simulink model "Sim_Multi"  (R2023a)
settings: Solver=FixedStepAuto  StartTime=0.0  StopTime=20  FixedStep=t_sim  MaxStep=t_control  RelTol=1e-5  EnableMultiTasking=on
InitFcn:
  | %--------------------------------------------------------------------------
  | %% Multirotor Dynamic Simulation Environment for the Testing of GNC Algorithms
  | % This simulation is part of the Master's thesis titled
  | % "A Modular Simulation Environment for the Improved Dynamic Simulation of
  | % Multirotor Unmanned Aerial Vehicles",
  | % submitted to the University of Illinois at Urbana-Champaign in May 2016.
  | % The thesis itself can be found here: http://hdl.handle.net/2142/90660
  | % Jan Vervoorst, vervoors@illinois.edu
  | % University of Illinois 2015/16
  | %--------------------------------------------------------------------------
  | %% Initialization routine for the Simulink simulation file Sim_Multi.slx
  | %--------------------------------------------------------------------------
  | clear all;close all;clc
  | %--------------------------------------------------------------------------
  | t_control = 1/500;          % Controller/state estimation frequency 500Hz [s]
  | t_sim = t_control/2;        % Simulation frequency 1000Hz [s]
  | sim_time = 10.0;            % Duration of simulation [sec]
  | r2d = 180/pi;               % Conversion factor radians to degrees [deg/rad]
  | d2r = pi/180;               % Conversion factor degrees to radians [rad/deg]
  | g = 9.80665;                % Acceleration of gravity [m/s^2]
  | rpm2radpersec = 2*pi/60;    % Conversion factor RPM to rad/sec [rad/(s*rpm)]
  | rho = 1.225;                % Density of air [kg/m^3]
  | %--------------------------------------------------------------------------
  | %%%%%%%%%%%%%%%%%%%%%%%%%%%%%%%%%%%%%%%%%%%%%%%%%%%%%%%%%%%%%%%%%%%%%%%%%%%
  | %               Quad specific configuration parameters                    %
  | %%%%%%%%%%%%%%%%%%%%%%%%%%%%%%%%%%%%%%%%%%%%%%%%%%%%%%%%%%%%%%%%%%%%%%%%%%%
  | % The coordinate system used in this model is defined as follows:
  | % X: pointing forward, Roll axis
  | % Y: pointing to the right, Pitch axis
  | % Z: pointing down, Yaw axis
  | % To define the geometry of the airframe, the following convention is used:
  | % - the base airframe is assumed to be somewhat symmetric
  | % - the CoG for the base airframe coincides with the geometric center in X/Y plane (but is shifted along Z axis)
  | % - the motor arm length in X/Y plane is defined as the distance to the geometric center of the base airframe
  | % - motor thrust is generated at the prop, which is offset a distance (along Z) from the geometric center
  | % - motor thrust vector may be misaligned from purely Z direction, so a set of rotation angles is given for each motor
  | % - real position of CoG is given as a position vector from geometric center
  | % - everything is expressed in body coordinate system described above
  | %%%%%%%%%%%%%%%%%%%%%%%%%%%%%%%%%%%%%%%%%%%%%%%%%%%%%%%%%%%%%%%%%%%%%%%%%%%
  | Noise_flag = 0;                 % Set to 1 for sensor/estimation noise, to 0 for no noise
  | Coriolis_correction = 1;        % Set to 1 to cancel omega x (J*omega) term in control law, 0 if not
  | Dyn_thrust = 1;                 % Set to 1 to engage dynamic thrust effects, to 0 to disengage
  | Blade_flapping = 1;             % Set to 1 to engage blade flapping effects, to 0 to disengage
  | %%%%%%%%%%%%%%%%%%%%%%%%%%%%%%%%
  | % Initial conditions
  | Att_init = [0;0;0] * d2r;       % Initial airframe attitude in Euler angles Roll/Pitch/Yaw for 6DOF block [deg]
  | omega_init = [0;0;0];           % Initial angular rates in Body frame for 6DOF block [rad/s]
  | Vb_init = [0;0;0];              % Initial velocity in Body frame for 6DOF block [m/s]
  | Xi_init = [0;0;0];              % Initial position in Inertial frame for 6DOF block [m]
  | rpm_init = 3104.5025852;        % Initial motor speed [rpm]
  | q_init = rpy2quat(Att_init);    % Compute the initial attitude quaternion
  | R_IB_init = rpy2rot(Att_init);  % Compute the initial rotation matrix R_IB
  | Vi_init = R_IB_init' * Vb_init; % Compute the initial velocity in Inertial axes
  | %%%%%%%%%%%%%%%%%%%%%%%%%%%%%%%%
  | % Parameters for aerodynamic drag computation
  | a = 0.060;                      % Surface area of airframe visible along the Body x axis [m^2]
  | b = 0.060;                      % Surface area of airframe visible along the Body y axis [m^2]
  | c = 0.060;                      % Surface area of airframe visible along the Body z axis [m^2]
  | C_D = 0.40;                     % Drag coefficient [dimensionless]
  | Surface_params = [a;b;c];       % Combine the surface area parameters
  | ... (+145 lines)
undefined symbols (not defined in the file or in its folder): DiscIntNeverNeededParam, rpy2quat, thrust2rpm
libraries: simulink x20
(part 4 of 4)

== system Sim_Multi/multirotor/Force//Moment computation/Forces and moments generated by spinning propellers/For Each Subsystem/Thrust//moment vector for each propeller (Body axes)/Compute dynamic motor thrust and moments/Dynamic thrust ratio/Flight modes of the propeller ==
  v_h : Inport
  v_c : Inport  Port=2
  Divide : Product  Inputs=*/  SampleTime=t_sim
  If : If  IfExpression=u1 >= 0  ElseIfExpressions=u1 >= -2  SampleTime=t_sim
  Merge : Merge  Inputs=3
  Normal working state vc/vh >= 0 : Subsystem  TreatAsAtomicUnit=on
  "Vortex ring state -2 <= vc/vh < 0 " : Subsystem  TreatAsAtomicUnit=on
  Windmill braking state vc/vh < -2 : Subsystem  TreatAsAtomicUnit=on
  v_i : Outport
  wires:
  Merge/1 -> v_i/1
  v_c/1 -> Windmill braking state vc/vh < -2/1(v_c), "Vortex ring state -2 <= vc/vh < 0 "/1(v_c), Normal working state vc/vh >= 0/1(v_c), Divide/1
  v_h/1 -> Divide/2
  Divide/1 -> If/1  "v_c/v_h"
  If/1 -> Normal working state vc/vh >= 0/Action
  Normal working state vc/vh >= 0/1(v_i) -> Merge/1
  "Vortex ring state -2 <= vc/vh < 0 "/1(v_i) -> Merge/2
  Windmill braking state vc/vh < -2/1(v_i) -> Merge/3
  If/2 -> "Vortex ring state -2 <= vc/vh < 0 "/Action
  If/3 -> Windmill braking state vc/vh < -2/Action

== system Sim_Multi/multirotor/Force//Moment computation/Forces and moments generated by spinning propellers/For Each Subsystem/Thrust//moment vector for each propeller (Body axes)/Compute dynamic motor thrust and moments/Gyroscopic torque/Cross Product ==
  u : Inport
  v : Inport  Port=2
  Subsystem : Subsystem
  Subsystem1 : Subsystem
  Sum : Sum  Inputs=+|-
  u x v : Outport
  wires:
  Sum/1 -> u x v/1
  u/1 -> Subsystem1/1(u), Subsystem/1(u)
  v/1 -> Subsystem1/2(v), Subsystem/2(v)
  Subsystem/1(Positive elements) -> Sum/1
  Subsystem1/1(Negative elements) -> Sum/2

== system Sim_Multi/multirotor/Force//Moment computation/Forces and moments generated by spinning propellers/For Each Subsystem/Thrust//moment vector for each propeller (Body axes)/Compute dynamic motor thrust and moments/Gyroscopic torque/Propeller moment of inertia ==
  note: This computes the approximate moment of inertia of a propeller given its mass and diameter.
      | It is the mean value of the disk approximation and the rod approximation for a spinning propeller.
  In1 : Inport
  Gain : Gain  Gain=0.5
  Gain1 : Gain  Gain=7/12
  Product7 : Product  Inputs=3
  Selector4 : Selector  InputPortWidth=17  IndexOptions=Index vector (dialog)  Indices=[16]  OutputSizes=1
  Selector5 : Selector  InputPortWidth=17  IndexOptions=Index vector (dialog)  Indices=[17]  OutputSizes=1
  Out1 : Outport
  wires:
  Selector5/1 -> Product7/3  "Propeller mass"
  Gain/1 -> Product7/2, Product7/1
  In1/1 -> Selector5/1, Selector4/1
  Selector4/1 -> Gain/1  "Propeller diameter"
  Gain1/1 -> Out1/1
  Product7/1 -> Gain1/1

== system Sim_Multi/multirotor/Force//Moment computation/Forces and moments generated by spinning propellers/For Each Subsystem/Thrust//moment vector for each propeller (Body axes)/Coordinate transformation Body to Motor axes/Rotation Matrix Body to Motor/Subsystem ==
  Euler : Inport
  Demux : Demux  Outputs=3
  Product : Product
  Terminator : Terminator
  Trigonometric Function1 : Trigonometry  Operator=cos
  Trigonometric Function3 : Trigonometry  Operator=cos
  R_11 : Outport
  wires:
  Euler/1 -> Demux/1
  Demux/1 -> Terminator/1  "phi"
  Demux/2 -> Trigonometric Function1/1  "theta"
  Demux/3 -> Trigonometric Function3/1  "psi"
  Trigonometric Function1/1 -> Product/1
  Trigonometric Function3/1 -> Product/2
  Product/1 -> R_11/1

== system Sim_Multi/multirotor/Force//Moment computation/Forces and moments generated by spinning propellers/For Each Subsystem/Thrust//moment vector for each propeller (Body axes)/Coordinate transformation Body to Motor axes/Rotation Matrix Body to Motor/Subsystem1 ==
  Euler : Inport
  Demux : Demux  Outputs=3
  Product : Product
  Terminator : Terminator
  Trigonometric Function1 : Trigonometry  Operator=cos
  Trigonometric Function3 : Trigonometry
  R_12 : Outport
  wires:
  Euler/1 -> Demux/1
  Demux/1 -> Terminator/1  "phi"
  Demux/2 -> Trigonometric Function1/1  "theta"
  Demux/3 -> Trigonometric Function3/1  "psi"
  Trigonometric Function1/1 -> Product/1
  Trigonometric Function3/1 -> Product/2
  Product/1 -> R_12/1

== system Sim_Multi/multirotor/Force//Moment computation/Forces and moments generated by spinning propellers/For Each Subsystem/Thrust//moment vector for each propeller (Body axes)/Coordinate transformation Body to Motor axes/Rotation Matrix Body to Motor/Subsystem2 ==
  Euler : Inport
  Demux : Demux  Outputs=3
  Gain : Gain  Gain=-1
  Terminator : Terminator
  Terminator1 : Terminator
  Trigonometric Function1 : Trigonometry
  R_13 : Outport
  wires:
  Euler/1 -> Demux/1
  Demux/1 -> Terminator/1  "phi"
  Demux/2 -> Trigonometric Function1/1  "theta"
  Demux/3 -> Terminator1/1  "psi"
  Trigonometric Function1/1 -> Gain/1
  Gain/1 -> R_13/1

== system Sim_Multi/multirotor/Force//Moment computation/Forces and moments generated by spinning propellers/For Each Subsystem/Thrust//moment vector for each propeller (Body axes)/Coordinate transformation Body to Motor axes/Rotation Matrix Body to Motor/Subsystem3 ==
  Euler : Inport
  Demux : Demux  Outputs=3
  Product : Product  Inputs=3
  Product1 : Product
  Sum : Sum  Inputs=|+-
  Trigonometric Function : Trigonometry
  Trigonometric Function1 : Trigonometry
  Trigonometric Function12 : Trigonometry
  Trigonometric Function3 : Trigonometry  Operator=cos
  Trigonometric Function5 : Trigonometry  Operator=cos
  R_21 : Outport
  wires:
  Euler/1 -> Demux/1
  Demux/2 -> Trigonometric Function1/1  "theta"
  Demux/3 -> Trigonometric Function/1, Trigonometric Function3/1  "psi"
  Trigonometric Function3/1 -> Product/3
  Trigonometric Function1/1 -> Product/2
  Demux/1 -> Trigonometric Function5/1, Trigonometric Function12/1  "phi"
  Trigonometric Function12/1 -> Product/1
  Trigonometric Function5/1 -> Product1/1
  Trigonometric Function/1 -> Product1/2
  Product/1 -> Sum/1
  Sum/1 -> R_21/1
  Product1/1 -> Sum/2

== system Sim_Multi/multirotor/Force//Moment computation/Forces and moments generated by spinning propellers/For Each Subsystem/Thrust//moment vector for each propeller (Body axes)/Coordinate transformation Body to Motor axes/Rotation Matrix Body to Motor/Subsystem4 ==
  Euler : Inport
  Demux1 : Demux  Outputs=3
  Product1 : Product  Inputs=3
  Product2 : Product
  Sum : Sum  Inputs=|++
  Trigonometric Function : Trigonometry  Operator=cos
  Trigonometric Function12 : Trigonometry
  Trigonometric Function2 : Trigonometry
  Trigonometric Function4 : Trigonometry
  Trigonometric Function5 : Trigonometry  Operator=cos
  R_22 : Outport
  wires:
  Euler/1 -> Demux1/1
  Demux1/2 -> Trigonometric Function2/1  "theta"
  Demux1/3 -> Trigonometric Function/1, Trigonometric Function4/1  "psi"
  Trigonometric Function4/1 -> Product1/3
  Trigonometric Function2/1 -> Product1/2
  Demux1/1 -> Trigonometric Function5/1, Trigonometric Function12/1  "phi"
  Trigonometric Function12/1 -> Product1/1
  Trigonometric Function5/1 -> Product2/1
  Trigonometric Function/1 -> Product2/2
  Product1/1 -> Sum/1
  Sum/1 -> R_22/1
  Product2/1 -> Sum/2

== system Sim_Multi/multirotor/Force//Moment computation/Forces and moments generated by spinning propellers/For Each Subsystem/Thrust//moment vector for each propeller (Body axes)/Coordinate transformation Body to Motor axes/Rotation Matrix Body to Motor/Subsystem5 ==
  Euler : Inport
  Demux : Demux  Outputs=3
  Product : Product
  Terminator : Terminator
  Trigonometric Function1 : Trigonometry  Operator=cos
  Trigonometric Function3 : Trigonometry
  R_23 : Outport
  wires:
  Euler/1 -> Demux/1
  Demux/2 -> Trigonometric Function1/1  "theta"
  Product/1 -> R_23/1
  Demux/1 -> Trigonometric Function3/1  "phi"
  Demux/3 -> Terminator/1  "psi"
  Trigonometric Function3/1 -> Product/1
  Trigonometric Function1/1 -> Product/2

== system Sim_Multi/multirotor/Force//Moment computation/Forces and moments generated by spinning propellers/For Each Subsystem/Thrust//moment vector for each propeller (Body axes)/Coordinate transformation Body to Motor axes/Rotation Matrix Body to Motor/Subsystem6 ==
  Euler : Inport
  Demux1 : Demux  Outputs=3
  Product1 : Product  Inputs=3
  Product2 : Product
  Sum : Sum  Inputs=|++
  Trigonometric Function : Trigonometry
  Trigonometric Function12 : Trigonometry  Operator=cos
  Trigonometric Function2 : Trigonometry
  Trigonometric Function4 : Trigonometry  Operator=cos
  Trigonometric Function5 : Trigonometry
  R_31 : Outport
  wires:
  Euler/1 -> Demux1/1
  Demux1/2 -> Trigonometric Function2/1  "theta"
  Demux1/3 -> Trigonometric Function/1, Trigonometric Function4/1  "psi"
  Trigonometric Function4/1 -> Product1/3
  Trigonometric Function2/1 -> Product1/2
  Demux1/1 -> Trigonometric Function5/1, Trigonometric Function12/1  "phi"
  Trigonometric Function12/1 -> Product1/1
  Trigonometric Function5/1 -> Product2/1
  Trigonometric Function/1 -> Product2/2
  Product1/1 -> Sum/1
  Sum/1 -> R_31/1
  Product2/1 -> Sum/2

== system Sim_Multi/multirotor/Force//Moment computation/Forces and moments generated by spinning propellers/For Each Subsystem/Thrust//moment vector for each propeller (Body axes)/Coordinate transformation Body to Motor axes/Rotation Matrix Body to Motor/Subsystem7 ==
  Euler : Inport
  Demux : Demux  Outputs=3
  Product : Product  Inputs=3
  Product1 : Product
  Sum : Sum  Inputs=|+-
  Trigonometric Function : Trigonometry  Operator=cos
  Trigonometric Function1 : Trigonometry
  Trigonometric Function12 : Trigonometry  Operator=cos
  Trigonometric Function3 : Trigonometry
  Trigonometric Function5 : Trigonometry
  R_32 : Outport
  wires:
  Euler/1 -> Demux/1
  Demux/2 -> Trigonometric Function1/1  "theta"
  Demux/3 -> Trigonometric Function/1, Trigonometric Function3/1  "psi"
  Trigonometric Function3/1 -> Product/3
  Trigonometric Function1/1 -> Product/2
  Demux/1 -> Trigonometric Function5/1, Trigonometric Function12/1  "phi"
  Trigonometric Function12/1 -> Product/1
  Trigonometric Function5/1 -> Product1/1
  Trigonometric Function/1 -> Product1/2
  Product/1 -> Sum/1
  Sum/1 -> R_32/1
  Product1/1 -> Sum/2

== system Sim_Multi/multirotor/Force//Moment computation/Forces and moments generated by spinning propellers/For Each Subsystem/Thrust//moment vector for each propeller (Body axes)/Coordinate transformation Body to Motor axes/Rotation Matrix Body to Motor/Subsystem8 ==
  Euler : Inport
  Demux : Demux  Outputs=3
  Product : Product
  Terminator : Terminator
  Trigonometric Function1 : Trigonometry  Operator=cos
  Trigonometric Function3 : Trigonometry  Operator=cos
  R_33 : Outport
  wires:
  Euler/1 -> Demux/1
  Demux/2 -> Trigonometric Function1/1  "theta"
  Product/1 -> R_33/1
  Demux/3 -> Terminator/1  "psi"
  Demux/1 -> Trigonometric Function3/1  "phi"
  Trigonometric Function3/1 -> Product/1
  Trigonometric Function1/1 -> Product/2

== system Sim_Multi/multirotor/Force//Moment computation/Forces and moments generated by spinning propellers/For Each Subsystem/Thrust//moment vector for each propeller (Body axes)/Coordinate transformation Body to Motor axes/Rotation Matrix Body to Motor/Subsystem9 ==
  R_11 : Inport  PortDimensions=1
  R_12 : Inport  Port=2  PortDimensions=1
  R_13 : Inport  Port=3  PortDimensions=1
  R_21 : Inport  Port=4  PortDimensions=1
  R_22 : Inport  Port=5  PortDimensions=1
  R_23 : Inport  Port=6  PortDimensions=1
  R_31 : Inport  Port=7  PortDimensions=1
  R_32 : Inport  Port=8  PortDimensions=1
  R_33 : Inport  Port=9  PortDimensions=1
  Reshape (9) to [3x3] column-major : Reshape  OutputDimensionality=Customize  OutputDimensions=[3,3]
  Vector Concatenate : Concatenate  NumInputs=9
  R_mb : Outport
  wires:
  R_33/1 -> Vector Concatenate/9
  R_22/1 -> Vector Concatenate/5
  Reshape (9) to [3x3] column-major/1 -> R_mb/1
  R_11/1 -> Vector Concatenate/1
  Vector Concatenate/1 -> Reshape (9) to [3x3] column-major/1
  R_32/1 -> Vector Concatenate/6
  R_31/1 -> Vector Concatenate/3
  R_21/1 -> Vector Concatenate/2
  R_13/1 -> Vector Concatenate/7
  R_12/1 -> Vector Concatenate/4
  R_23/1 -> Vector Concatenate/8

== system Sim_Multi/multirotor/Force//Moment computation/Compute aerodynamic drag of the airframe in Body axes/Aerodynamic drag force/Nonzero airspeed/Surface area computation/Surface area computation/norm/dot_product ==
  u : Inport
  v : Inport  Port=2
  Product : Product  Multiplication=Matrix(*)  RndMeth=Zero
  Reshape : Reshape  OutputDimensionality=Column vector (2-D)
  Reshape1 : Reshape  OutputDimensionality=Column vector (2-D)
  transpose : Math  Operator=transpose  SignedPower=on
  u.v : Outport
  wires:
  v/1 -> Reshape1/1
  u/1 -> Reshape/1
  Reshape/1 -> transpose/1
  transpose/1 -> Product/1
  Reshape1/1 -> Product/2
  Product/1 -> u.v/1

== system Sim_Multi/multirotor/Force//Moment computation/Forces and moments generated by spinning propellers/For Each Subsystem/Thrust//moment vector for each propeller (Body axes)/Compute dynamic motor thrust and moments/Blade flapping computations/Nonzero airspeed in rotor plane/norm ==
  u : Inport
  Complex to Real-Imag : ComplexToRealImag  Output=Real
  Sqrt : Sqrt
  dot_product : Subsystem
  ||u|| : Outport
  wires:
  u/1 -> dot_product/1(u), dot_product/2(v)
  dot_product/1(u.v) -> Sqrt/1
  Sqrt/1 -> Complex to Real-Imag/1
  Complex to Real-Imag/1 -> ||u||/1

== system Sim_Multi/multirotor/Force//Moment computation/Forces and moments generated by spinning propellers/For Each Subsystem/Thrust//moment vector for each propeller (Body axes)/Compute dynamic motor thrust and moments/Blade flapping computations/norm/dot_product ==
  u : Inport
  v : Inport  Port=2
  Product : Product  Multiplication=Matrix(*)  RndMeth=Zero
  Reshape : Reshape  OutputDimensionality=Column vector (2-D)
  Reshape1 : Reshape  OutputDimensionality=Column vector (2-D)
  transpose : Math  Operator=transpose  SignedPower=on
  u.v : Outport
  wires:
  v/1 -> Reshape1/1
  u/1 -> Reshape/1
  Reshape/1 -> transpose/1
  transpose/1 -> Product/1
  Reshape1/1 -> Product/2
  Product/1 -> u.v/1

== system Sim_Multi/multirotor/Force//Moment computation/Forces and moments generated by spinning propellers/For Each Subsystem/Thrust//moment vector for each propeller (Body axes)/Compute dynamic motor thrust and moments/Dynamic thrust ratio/Angle of attack and airspeed magnitude/Nonzero airspeed ==
  Airspeed (Motor) : Inport
  Action Port : ActionPort  ActionPortLabel=else
  Demux : Demux  Outputs=[2,1]
  Divide1 : Product  Inputs=/*
  Trigonometric Function : Trigonometry  Operator=atan
  norm1 : Subsystem
  AoA (rad) : Outport
  wires:
  Trigonometric Function/1 -> AoA (rad)/1
  Demux/1 -> norm1/1(u)  "Airspeed xy component"
  Demux/2 -> Divide1/2  "Airspeed z component"
  norm1/1(||u||) -> Divide1/1
  Divide1/1 -> Trigonometric Function/1
  Airspeed (Motor)/1 -> Demux/1

== system Sim_Multi/multirotor/Force//Moment computation/Forces and moments generated by spinning propellers/For Each Subsystem/Thrust//moment vector for each propeller (Body axes)/Compute dynamic motor thrust and moments/Dynamic thrust ratio/Angle of attack and airspeed magnitude/Zero airspeed ==
  Airspeed (Motor) : Inport
  Action Port : ActionPort  ActionPortLabel=if(u1 == 0)
  Constant : Constant  Value=0
  Terminator : Terminator
  AoA (rad) : Outport  InitialOutput=[0]
  wires:
  Airspeed (Motor)/1 -> Terminator/1  "Airspeed (Motor axes)"
  Constant/1 -> AoA (rad)/1

== system Sim_Multi/multirotor/Force//Moment computation/Forces and moments generated by spinning propellers/For Each Subsystem/Thrust//moment vector for each propeller (Body axes)/Compute dynamic motor thrust and moments/Dynamic thrust ratio/Angle of attack and airspeed magnitude/norm2 ==
  u : Inport
  Complex to Real-Imag : ComplexToRealImag  Output=Real
  Sqrt : Sqrt
  dot_product : Subsystem
  ||u|| : Outport
  wires:
  u/1 -> dot_product/1(u), dot_product/2(v)
  dot_product/1(u.v) -> Sqrt/1
  Sqrt/1 -> Complex to Real-Imag/1
  Complex to Real-Imag/1 -> ||u||/1

== system Sim_Multi/multirotor/Force//Moment computation/Forces and moments generated by spinning propellers/For Each Subsystem/Thrust//moment vector for each propeller (Body axes)/Compute dynamic motor thrust and moments/Dynamic thrust ratio/Flight modes of the propeller/Normal working state vc//vh >= 0 ==
  v_c : Inport
  Action Port : ActionPort  ActionPortLabel=if(u1 >= 0)
  Gain : Gain  Gain=0.5
  Induced velocity at hover : Constant  Value=v_h
  Product : Product
  Product1 : Product
  Sqrt : Sqrt
  Sum : Sum  Inputs=|-+
  Sum1 : Sum  Inputs=|++
  v_i : Outport
  wires:
  v_c/1 -> Gain/1  "Climb velocity"
  Gain/1 -> Product/2, Product/1, Sum/1
  Sqrt/1 -> Sum/2
  Sum/1 -> v_i/1
  Product/1 -> Sum1/1
  Sum1/1 -> Sqrt/1
  Induced velocity at hover/1 -> Product1/2, Product1/1
  Product1/1 -> Sum1/2

== system Sim_Multi/multirotor/Force//Moment computation/Forces and moments generated by spinning propellers/For Each Subsystem/Thrust//moment vector for each propeller (Body axes)/Compute dynamic motor thrust and moments/Dynamic thrust ratio/Flight modes of the propeller/Vortex ring state -2 <= vc//vh < 0  ==
  v_c : Inport
  Action Port : ActionPort  ActionPortLabel=elseif(u1 >= -2)
  Add : Sum  Inputs=+++++
  Constant : Constant  Value=kappa
  Divide : Product  Inputs=*/
  Gain : Gain  Gain=k1
  Gain1 : Gain  Gain=k2
  Gain2 : Gain  Gain=k3
  Gain3 : Gain  Gain=k4
  Induced velocity at hover : Constant  Value=v_h
  Product{,1..3} (4 alike) : Product
  v_i : Outport
  wires:
  v_c/1 -> Divide/1  "Climb velocity"
  Induced velocity at hover/1 -> Product3/2, Divide/2
  Divide/1 -> Product2/2, Product1/2, Product/2, Product/1, Gain/1
  Product/1 -> Gain1/1, Product1/1
  Product1/1 -> Gain2/1, Product2/1
  Product2/1 -> Gain3/1
  Gain3/1 -> Add/5
  Gain2/1 -> Add/4
  Gain1/1 -> Add/3
  Gain/1 -> Add/2
  Constant/1 -> Add/1
  Add/1 -> Product3/1
  Product3/1 -> v_i/1

== system Sim_Multi/multirotor/Force//Moment computation/Forces and moments generated by spinning propellers/For Each Subsystem/Thrust//moment vector for each propeller (Body axes)/Compute dynamic motor thrust and moments/Dynamic thrust ratio/Flight modes of the propeller/Windmill braking state vc//vh < -2 ==
  v_c : Inport
  Action Port : ActionPort  ActionPortLabel=else
  Gain : Gain  Gain=0.5
  Induced velocity at hover : Constant  Value=v_h
  Product : Product
  Product1 : Product
  Sqrt : Sqrt
  Sum : Sum  Inputs=|--
  Sum1 : Sum  Inputs=|+-
  v_i : Outport
  wires:
  v_c/1 -> Gain/1  "Climb velocity"
  Gain/1 -> Product/2, Product/1, Sum/1
  Sqrt/1 -> Sum/2
  Sum/1 -> v_i/1
  Product/1 -> Sum1/1
  Sum1/1 -> Sqrt/1
  Induced velocity at hover/1 -> Product1/2, Product1/1
  Product1/1 -> Sum1/2

== system Sim_Multi/multirotor/Force//Moment computation/Forces and moments generated by spinning propellers/For Each Subsystem/Thrust//moment vector for each propeller (Body axes)/Compute dynamic motor thrust and moments/Gyroscopic torque/Cross Product/Subsystem ==
  u : Inport
  v : Inport  Port=2
  Demux : Demux  Outputs=3
  Demux1 : Demux  Outputs=3
  Mux : Mux  Inputs=3
  Product : Product
  Product1 : Product
  Product2 : Product
  Positive elements : Outport
  wires:
  Mux/1 -> Positive elements/1
  v/1 -> Demux1/1
  u/1 -> Demux/1
  Demux/2 -> Product/1
  Demux1/3 -> Product/2
  Demux/3 -> Product1/1
  Demux1/1 -> Product1/2
  Demux/1 -> Product2/1
  Demux1/2 -> Product2/2
  Product/1 -> Mux/1
  Product1/1 -> Mux/2
  Product2/1 -> Mux/3

== system Sim_Multi/multirotor/Force//Moment computation/Forces and moments generated by spinning propellers/For Each Subsystem/Thrust//moment vector for each propeller (Body axes)/Compute dynamic motor thrust and moments/Gyroscopic torque/Cross Product/Subsystem1 ==
  u : Inport
  v : Inport  Port=2
  Demux : Demux  Outputs=3
  Demux1 : Demux  Outputs=3
  Mux : Mux  Inputs=3
  Product : Product
  Product1 : Product
  Product2 : Product
  Negative elements : Outport
  wires:
  Mux/1 -> Negative elements/1
  v/1 -> Demux1/1
  u/1 -> Demux/1
  Product/1 -> Mux/1
  Product1/1 -> Mux/2
  Product2/1 -> Mux/3
  Demux/3 -> Product/1
  Demux1/2 -> Product/2
  Demux/1 -> Product1/1
  Demux1/3 -> Product1/2
  Demux/2 -> Product2/1
  Demux1/1 -> Product2/2

== system Sim_Multi/multirotor/Force//Moment computation/Forces and moments generated by spinning propellers/For Each Subsystem/Thrust//moment vector for each propeller (Body axes)/Compute dynamic motor thrust and moments/Blade flapping computations/Nonzero airspeed in rotor plane/norm/dot_product ==
  u : Inport
  v : Inport  Port=2
  Product : Product  Multiplication=Matrix(*)  RndMeth=Zero
  Reshape : Reshape  OutputDimensionality=Column vector (2-D)
  Reshape1 : Reshape  OutputDimensionality=Column vector (2-D)
  transpose : Math  Operator=transpose  SignedPower=on
  u.v : Outport
  wires:
  v/1 -> Reshape1/1
  u/1 -> Reshape/1
  Reshape/1 -> transpose/1
  transpose/1 -> Product/1
  Reshape1/1 -> Product/2
  Product/1 -> u.v/1

== system Sim_Multi/multirotor/Force//Moment computation/Forces and moments generated by spinning propellers/For Each Subsystem/Thrust//moment vector for each propeller (Body axes)/Compute dynamic motor thrust and moments/Dynamic thrust ratio/Angle of attack and airspeed magnitude/Nonzero airspeed/norm1 ==
  u : Inport
  Complex to Real-Imag : ComplexToRealImag  Output=Real
  Sqrt : Sqrt
  dot_product : Subsystem
  ||u|| : Outport
  wires:
  u/1 -> dot_product/1(u), dot_product/2(v)
  dot_product/1(u.v) -> Sqrt/1
  Sqrt/1 -> Complex to Real-Imag/1
  Complex to Real-Imag/1 -> ||u||/1

== system Sim_Multi/multirotor/Force//Moment computation/Forces and moments generated by spinning propellers/For Each Subsystem/Thrust//moment vector for each propeller (Body axes)/Compute dynamic motor thrust and moments/Dynamic thrust ratio/Angle of attack and airspeed magnitude/norm2/dot_product ==
  u : Inport
  v : Inport  Port=2
  Product : Product  Multiplication=Matrix(*)  RndMeth=Zero
  Reshape : Reshape  OutputDimensionality=Column vector (2-D)
  Reshape1 : Reshape  OutputDimensionality=Column vector (2-D)
  transpose : Math  Operator=transpose  SignedPower=on
  u.v : Outport
  wires:
  v/1 -> Reshape1/1
  u/1 -> Reshape/1
  Reshape/1 -> transpose/1
  transpose/1 -> Product/1
  Reshape1/1 -> Product/2
  Product/1 -> u.v/1

== system Sim_Multi/multirotor/Force//Moment computation/Forces and moments generated by spinning propellers/For Each Subsystem/Thrust//moment vector for each propeller (Body axes)/Compute dynamic motor thrust and moments/Dynamic thrust ratio/Angle of attack and airspeed magnitude/Nonzero airspeed/norm1/dot_product ==
  u : Inport
  v : Inport  Port=2
  Product : Product  Multiplication=Matrix(*)  RndMeth=Zero
  Reshape : Reshape  OutputDimensionality=Column vector (2-D)
  Reshape1 : Reshape  OutputDimensionality=Column vector (2-D)
  transpose : Math  Operator=transpose  SignedPower=on
  u.v : Outport
  wires:
  v/1 -> Reshape1/1
  u/1 -> Reshape/1
  Reshape/1 -> transpose/1
  transpose/1 -> Product/1
  Reshape1/1 -> Product/2
  Product/1 -> u.v/1

== matlab function Sim_Multi/multirotor/6DOF model/Quat Strapdown Eq./MATLAB Function ==
  data: quat_input input; quat_output output
% Jan Vervoorst, vervoors@illinois.edu
% University of Illinois 2015/16
%--------------------------------------------------------------------------
%% Find quaternion from roll, pitch, yaw
%  This files takes Roll/Pitch/Yaw Euler angles as inputs
% and transforms into the quaternion representation.
% Representative of Euler angle sequence (1,2,3) according to
% "Representing Attitude: Euler Angles, Unit Quaternions, and Rotation Vectors"
% by James Diebel, Stanford University, 20 October 2006
%--------------------------------------------------------------------------
function quat_output = rpy2quat(quat_input)
%-------------------------------------------------------
% System states
roll  = quat_input(1);  % Roll input [rad]
pitch = quat_input(2);  % Pitch input [rad]
yaw   = quat_input(3);  % Yaw input [rad]
%-------------------------------------------------------
phi   = roll / 2;
theta = pitch / 2;
psi   = yaw / 2;
%
cphi   = cos(phi);
sphi   = sin(phi);
ctheta = cos(theta);
stheta = sin(theta);
cpsi   = cos(psi);
spsi   = sin(psi);
%
% This is the (1,2,3) angle sequence computation:
q0 = cphi * ctheta * cpsi + sphi * stheta * spsi;
q1 = sphi * ctheta * cpsi - cphi * stheta * spsi;
q2 = cphi * stheta * cpsi + sphi * ctheta * spsi;
q3 = cphi * ctheta * spsi - sphi * stheta * cpsi;
%-------------------------------------------------------	
if (q0 < 0.0)       % q0 always positive for uniqueness of the quaternion
    q0 = -q0;
	q1 = -q1;
	q2 = -q2;
	q3 = -q3;
end
%-------------------------------------------------------
% Outputs are the four entries of the desired normalized attitude quaternion
quat_output = [0 0 0 0]';
quat_output(1,1) = q0;
quat_output(2,1) = q1;
quat_output(3,1) = q2;
quat_output(4,1) = q3;
%--------------------------------------------------------------------------
% end of file

== matlab function Sim_Multi/Controller/Mapping thrust to rpm and saturation/For Each Subsystem/MATLAB Function ==
  data: thrust_input input; rpm_output output
% Jan Vervoorst, vervoors@illinois.edu
% University of Illinois 2015/16
%--------------------------------------------------------------------------
%% Compute desired motor rpm from thrust command
% Using a nominal second order model of the thrust equation, compute the
% desired motor RPM from a commanded thrust input.
%--------------------------------------------------------------------------
function rpm_output = thrust2rpm(thrust_input)
%-------------------------------------------------------
% System states
a1     = thrust_input(1);  % Linear thrust parameter a1
a2     = thrust_input(2);  % Quadratic thrust parameter a2
thrust = thrust_input(3);  % Desired thrust command
%-------------------------------------------------------
% Motor RPM and thrust are related by a quadratic function of the form
% thrust = a1 * RPM + a2 * RPM^2
% This quadratic equation is then solved for the RPM value
% (and only the positive solution is considered):
rpm_output = -a1/(2*a2) + sqrt((a1/(2*a2))^2 + thrust/a2);
%--------------------------------------------------------------------------
% end of file

== matlab function Sim_Multi/multirotor/Disturbances & Dynamic Events/MATLAB Function ==
  data: MotorMatrix_real output; arm_length input; arm_radius input; Motor_arm_angle input; prop_height input; prop_diameter input; rotation_direction input; max_rpm input; min_rpm input; COM_system output; total_mass output; inertial_matrix output; Surface_params output; mass_center input; COM_mass_center input; Surface_params_in input
function [MotorMatrix_real, COM_system, total_mass, inertial_matrix, Surface_params]= motor_matrix(arm_length, arm_radius , Motor_arm_angle, prop_height, prop_diameter,rotation_direction, max_rpm, min_rpm, mass_center, COM_mass_center, Surface_params_in)

%%%%%%%%%%%%%%%%%%%%%%%%%%%%%%%%
% MotorMatrix_real holds all the information about the actual performance
% of each actuator. The data is arranged as one row per motor/prop combo:
% 1      : Motor arm angle measured clockwise (looking from above) from the positive X axis (forward direction) [deg]
% 2      : Distance of prop/motor in X/Y plane from the geometric center of the airframe [m]
% 3      : Distance of prop/motor in Z direction from the geometric center of the airframe [m]
% 4      : Direction of prop rotation: -1 for CW, +1 for CCW [unitless]
% 5      : Control effectiveness of the actuator (nominally 1.0)
% 6      : First-order motor transfer function time constant [sec]
% 7..8   : Two coefficients that describe the RPM to thrust [N] transfer function for static conditions [a1 a2]
%          Thrust = a1 * RPM + a2 * RPM^2
% 9..10  : Two coefficients that describe the RPM to torque [Nm] transfer function for static conditions [b1 b2]
%          Torque = b1 * RPM + b2 * RPM^2
% 11     : Minimum RPM value of the actuator
% 12     : Maximum RPM value of the actuator
% 13..15 : Rotations of thrust vector around Body-fixed axes away from nominal direction [deg]
%          Nominal direction of thrust vector is [0;0;-1]
%          Rotation order from body to motor axes is Yaw/Pitch/Roll (Euler angle sequence (1,2,3))
% 16     : Propeller diameter [m]
% 17     : Propeller mass [kg]
 
Surface_params = Surface_params_in;
Rz = zeros(3, 3, 4);
Motor_arm_angle_rad = [45 135 225 315] * pi/180; 

for i = 1:4
   Rz(:,:,i) = [cos(Motor_arm_angle_rad(i)) -sin(Motor_arm_angle_rad(i)) 0; sin(Motor_arm_angle_rad(i)) cos(Motor_arm_angle_rad(i)) 0; 0 0 1];
end

propeller_mass = prop_diameter .* (0.0110/ 0.2032);
total_propeller_mass = sum(propeller_mass);

volume = pi .* arm_length .* arm_radius.^2;
airframe_mass = 1700 * volume;
total_airframe_mass = sum(airframe_mass);

total_mass = mass_center + total_airframe_mass + total_propeller_mass;

COM_propeller = zeros(4, 3);
COM_airframe = zeros(4, 3);

for i = 1:4
    COM_propeller(i,:) = Rz(:,:,i) * [arm_length(i) 0 prop_height(i)]';
    COM_airframe(i,:) = Rz(:,:,i) * [arm_length(i)/2 0 0]';
end

% Computing the weighted sum for center of mass
COM_propeller_total = [sum(propeller_mass' .* COM_propeller(:,1)); sum(propeller_mass' .* COM_propeller(:,2)); sum(propeller_mass' .* COM_propeller(:,3))];
COM_airframe_total = [sum(airframe_mass' .* COM_airframe(:,1)); sum(airframe_mass' .* COM_airframe(:,2)); sum(airframe_mass' .* COM_airframe(:,3))];
COM_center_total = mass_center .* COM_mass_center';  

COM_system_inter = (COM_propeller_total(:,1) + COM_airframe_total(:,1) + COM_center_total) / (total_propeller_mass + total_airframe_mass + mass_center);
COM_system = COM_system_inter(:,1);
% Inertia calculation
I_total = zeros(3, 3);

% ... [previous code]

for i = 1:4
    % Propeller
    I_propeller_cm = diag([1/12*propeller_mass(i)*arm_length(i)^2, 1/12*propeller_mass(i)*arm_length(i)^2, 0]);
    d_propeller = COM_propeller(i,:)' - COM_system; 
    
    d_propeller_outer_product = d_propeller * d_propeller'; 
    scalar_part = propeller_mass(i) * dot(d_propeller, d_propeller);
    I_propeller_total = I_propeller_cm + scalar_part .* eye(3) - propeller_mass(i) * d_propeller_outer_product;
    
    % Airframe
    I_cylinder_longitudinal = 1/2 * airframe_mass(i) * arm_radius(i)^2;
    I_cylinder_perpendicular = 1/4 * airframe_mass(i) * arm_radius(i)^2 + 1/12 * airframe_mass(i) * arm_length(i)^2;
    I_airframe_cm = diag([I_cylinder_perpendicular, I_cylinder_perpendicular, I_cylinder_longitudinal]);
    d_airframe = COM_airframe(i,:)' - COM_system;
    
    d_airframe_outer_product = d_airframe * d_airframe'; 
    scalar_part_airframe = airframe_mass(i) * dot(d_airframe, d_airframe);
    I_airframe_total = I_airframe_cm + scalar_part_airframe .* eye(3) - airframe_mass(i) * d_airframe_outer_product;
    
end
inertial_matrix_inter = diag(I_total + I_propeller_total + I_airframe_total);
% inertial_matrix = I_total + I_propeller_total + I_airframe_total;
% disp(inertial_matrix)

inertial_matrix = [inertial_matrix_inter(1) 0 0;
                    0 inertial_matrix_inter(2) 0;
                    0 0 inertial_matrix_inter(3)];

MotorMatrix_real = [Motor_arm_angle(1) , arm_length(1) , prop_height(1) , rotation_direction(1) , 1.0 , 0.010 , [9.6820 , 0.010872]*1e-5 , [1.4504 , 0.0016312]*1e-6 , min_rpm(1) , max_rpm(1) , [0.0 , 0.0 , 0.0] , prop_diameter(1) , propeller_mass(1); ...
                    Motor_arm_angle(2) , arm_length(2) , prop_height(2) , rotation_direction(2) , 1.0 , 0.010 , [9.6820 , 0.010872]*1e-5 , [1.4504 , 0.0016312]*1e-6 , min_rpm(2) , max_rpm(2) , [0.0 , 0.0 , 0.0] , prop_diameter(2) , propeller_mass(2); ...
                    Motor_arm_angle(3) , arm_length(3) , prop_height(3) , rotation_direction(3) , 1.0 , 0.010 , [9.6820 , 0.010872]*1e-5 , [1.4504 , 0.0016312]*1e-6 , min_rpm(3) , max_rpm(3) , [0.0 , 0.0 , 0.0] , prop_diameter(3) , propeller_mass(3); ...
                    Motor_arm_angle(4) , arm_length(4) , prop_height(4) , rotation_direction(4) , 1.0 , 0.010 , [9.6820 , 0.010872]*1e-5 , [1.4504 , 0.0016312]*1e-6 , min_rpm(4) , max_rpm(4) , [0.0 , 0.0 , 0.0] , prop_diameter(4) , propeller_mass(4)];
